simulink model "CONTROLADORES"  (R2018b)
settings: Solver=VariableStepAuto  StartTime=0.0  StopTime=8  RelTol=1e-3
undefined symbols (not defined in the file or in its folder): DiscIntNeverNeededParam, Gp, Gp_ps, M1p, magnitude, PID_Z, PIDM1z, Ts
libraries: simulink x3
settings Model: Creator=Vflrz17  LastModifiedBy=Atomauro
settings SFSimCC: SimUseLocalCustomCode=off
settings RTWCC: RTWUseLocalCustomCode=off

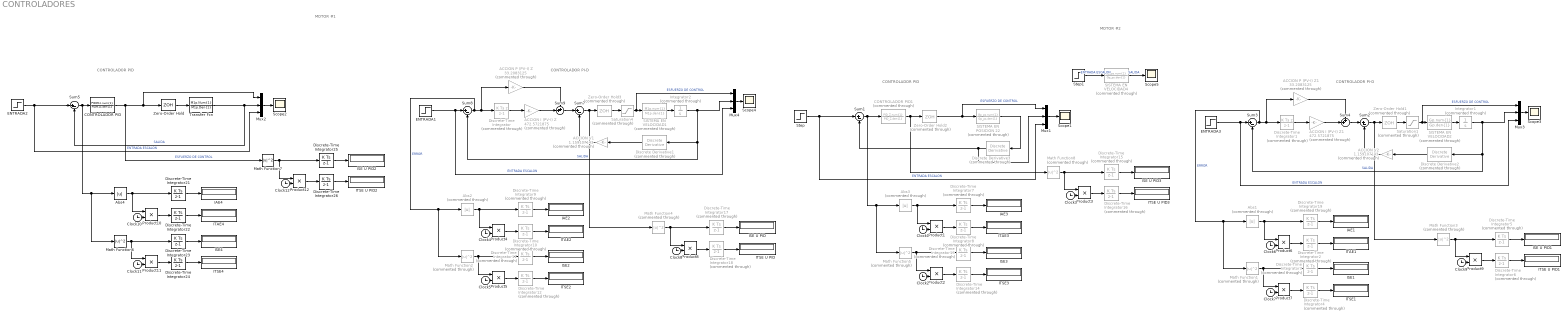
== system CONTROLADORES ==
  note: MOTOR #1
  note: CONTROLADOR PID
  note: CONTROLADOR PI-D
  note: MOTOR #2
  note: CONTROLADOR PID
  note: CONTROLADOR PI-D
  ACCION I (PV-I) Z : Gain  Commented=through  Gain=472.5721875
  ACCION I (PV-I) Z1 : Gain  Commented=through  Gain=472.5721875
  ACCION P (PV-I) Z : Gain  Commented=through  Gain=33.2083125
  ACCION P (PV-I) Z1 : Gain  Commented=through  Gain=33.2083125
  ACCION V1 : Gain  Commented=through  Gain=1.159107143
  ACCION V2 : Gain  Commented=through  Gain=1.159107143
  Abs1 : Abs  Commented=through
  Abs2 : Abs  Commented=through
  Abs3 : Abs  Commented=through
  Abs4 : Abs
  CONTROLADOR PID : DiscreteTransferFcn  Numerator=PIDM1z.num{1}  Denominator=PIDM1z.den{1}  SampleTime=Ts
  CONTROLADOR PID1 : DiscreteTransferFcn  Commented=through  Numerator=PID_Z.num{1}  Denominator=PID_Z.den{1}  SampleTime=Ts
  Clock{1..12} (12 alike) : Clock
  Discrete Derivative1 : simulink/Discrete/Discrete Derivative  Commented=through  gainval=1.0  ICPrevScaledInput=0.0  OutMin=[]  OutMax=[]  OutDataType=fixdt(1, 16)  OutScaling=2^-10  DoSatur=off
  Discrete Derivative2 : simulink/Discrete/Discrete Derivative  Commented=through  gainval=1.0  ICPrevScaledInput=0.0  OutMin=[]  OutMax=[]  OutDataType=fixdt(1, 16)  OutScaling=2^-10  DoSatur=off
  Discrete Derivative3 : simulink/Discrete/Discrete Derivative  Commented=through  gainval=1.0  ICPrevScaledInput=0.0  OutMin=[]  OutMax=[]  OutDataType=fixdt(1, 16)  OutScaling=2^-10  DoSatur=off
  Discrete-Time Integrator : DiscreteIntegrator  Commented=through  IntegratorMethod=Integration: Backward Euler  gainval=1  SampleTime=0.1  ICPrevOutput=DiscIntNeverNeededParam  ICPrevScaledInput=DiscIntNeverNeededParam
  Discrete-Time Integrator1 : DiscreteIntegrator  Commented=through  IntegratorMethod=Integration: Backward Euler  gainval=1  SampleTime=0.1  ICPrevOutput=DiscIntNeverNeededParam  ICPrevScaledInput=DiscIntNeverNeededParam
  Discrete-Time Integrator{2..19} (18 alike) : DiscreteIntegrator  Commented=through  gainval=1  SampleTime=Ts  ICPrevOutput=DiscIntNeverNeededParam  ICPrevScaledInput=DiscIntNeverNeededParam
  Discrete-Time Integrator{21..26} (6 alike) : DiscreteIntegrator  gainval=1  SampleTime=Ts  ICPrevOutput=DiscIntNeverNeededParam  ICPrevScaledInput=DiscIntNeverNeededParam
  ENTRADA1 : Step  SampleTime=0
  ENTRADA2 : Step  SampleTime=0
  ENTRADA3 : Step  SampleTime=Ts
  IAE{1..4} (4 alike) : Display
  ISE U PID{,1..3} (4 alike) : Display
  ISE{1..4} (4 alike) : Display
  ITAE{1..4} (4 alike) : Display
  ITSE U PID{,1..3} (4 alike) : Display
  ITSE{1..4} (4 alike) : Display
  Integrator1 : Integrator  Commented=through
  Integrator2 : Integrator  Commented=through
  Math Function{1..5,8} (6 alike) : Math  Commented=through  Operator=magnitude^2  SaturateOnIntegerOverflow=on
  Math Function6 : Math  Operator=magnitude^2  SaturateOnIntegerOverflow=on
  Math Function7 : Math  Operator=magnitude^2  SaturateOnIntegerOverflow=on
  Mux{1..4} (4 alike) : Mux  Inputs=3
  Product{1..12} (12 alike) : Product
  SISTEMA EN POSICION 22 : TransferFcn  Commented=through  Numerator=Gp_ps.num{1}  Denominator=Gp_ps.den{1}
  SISTEMA EN VELOCIDAD1 : TransferFcn  Commented=through  Numerator=M1p.num{1}  Denominator=M1p.den{1}
  SISTEMA EN VELOCIDAD2 : TransferFcn  Commented=through  Numerator=Gp.num{1}  Denominator=Gp.den{1}
  SISTEMA EN VELOCIDAD4 : TransferFcn  Commented=through  Numerator=Gp_ps.num{1}  Denominator=Gp_ps.den{1}
  Saturation1 : Saturate  Commented=through  UpperLimit=10  LowerLimit=-10
  Saturation4 : Saturate  Commented=through  UpperLimit=10  LowerLimit=-10
  Scope{1..5} (5 alike) : Scope
  Step : Step  SampleTime=0
  Step1 : Step  SampleTime=0
  Sum{1..3,5,7..8} (6 alike) : Sum  Inputs=|+-
  Sum4 : Sum  Inputs=++|
  Sum9 : Sum  Inputs=++|
  Transfer Fcn : TransferFcn  Numerator=M1p.Num{1}  Denominator=M1p.Den{1}
  Zero-Order Hold : ZeroOrderHold  SampleTime=-1
  Zero-Order Hold1 : ZeroOrderHold  Commented=through  SampleTime=Ts
  Zero-Order Hold2 : ZeroOrderHold  Commented=through  SampleTime=Ts
  Zero-Order Hold3 : ZeroOrderHold  Commented=through  SampleTime=-1
  wires:
  Mux2/1 -> Scope2/1
  ENTRADA2/1 -> Sum5/1, Mux2/3  "ENTRADA ESCALON"
  Transfer Fcn/1 -> Sum5/2, Mux2/2  "SALIDA"
  CONTROLADOR PID/1 -> Zero-Order Hold/1, Mux2/1, Math Function7/1  "ESFUERZO DE CONTROL"
  Clock12/1 -> Product12/2
  Product12/1 -> Discrete-Time Integrator26/1
  Discrete-Time Integrator24/1 -> ITSE4/1
  Discrete-Time Integrator26/1 -> ITSE U PID2/1
  Math Function7/1 -> Discrete-Time Integrator25/1, Product12/1
  Discrete-Time Integrator25/1 -> ISE U PID2/1
  Abs4/1 -> Product10/1, Discrete-Time Integrator21/1
  Discrete-Time Integrator21/1 -> IAE4/1
  Product11/1 -> Discrete-Time Integrator24/1
  Clock10/1 -> Product10/2
  Sum5/1 -> Abs4/1, Math Function6/1, CONTROLADOR PID/1
  Discrete-Time Integrator22/1 -> ITAE4/1
  Product10/1 -> Discrete-Time Integrator22/1
  Math Function6/1 -> Discrete-Time Integrator23/1, Product11/1
  Clock11/1 -> Product11/2
  Discrete-Time Integrator23/1 -> ISE4/1
  Discrete-Time Integrator12/1 -> ITSE2/1
  Clock5/1 -> Product5/2
  Sum8/1 -> Abs2/1, Math Function2/1, Discrete-Time Integrator/1, ACCION P (PV-I) Z/1  "ERROR"
  Product8/1 -> Discrete-Time Integrator18/1
  Saturation4/1 -> Mux4/1, SISTEMA EN VELOCIDAD1/1  "ESFUERZO DE CONTROL"
  Abs2/1 -> Product4/1, Discrete-Time Integrator9/1
  Mux4/1 -> Scope4/1
  Sum7/1 -> Math Function4/1, Zero-Order Hold3/1
  ACCION P (PV-I) Z/1 -> Sum9/1
  ENTRADA1/1 -> Mux4/3, Sum8/1  "ENTRADA ESCALON"
  Discrete Derivative1/1 -> ACCION V1/1
  Sum9/1 -> Sum7/1
  Product4/1 -> Discrete-Time Integrator10/1
  SISTEMA EN VELOCIDAD1/1 -> Integrator2/1
  Discrete-Time Integrator18/1 -> ITSE U PID/1
  Integrator2/1 -> Mux4/2, Discrete Derivative1/1, Sum8/2  "SALIDA"
  Discrete-Time Integrator9/1 -> IAE2/1
  ACCION I (PV-I) Z/1 -> Sum9/2
  Math Function2/1 -> Discrete-Time Integrator11/1, Product5/1
  ACCION V1/1 -> Sum7/2
  Discrete-Time Integrator10/1 -> ITAE2/1
  Discrete-Time Integrator17/1 -> ISE U PID/1
  Clock8/1 -> Product8/2
  Product5/1 -> Discrete-Time Integrator12/1
  Clock4/1 -> Product4/2
  Discrete-Time Integrator11/1 -> ISE2/1
  Zero-Order Hold3/1 -> Saturation4/1
  Math Function4/1 -> Discrete-Time Integrator17/1, Product8/1
  Discrete-Time Integrator/1 -> ACCION I (PV-I) Z/1
  Discrete-Time Integrator1/1 -> ACCION I (PV-I) Z1/1
  Math Function3/1 -> Product9/1, Discrete-Time Integrator5/1
  Zero-Order Hold1/1 -> Saturation1/1
  Discrete-Time Integrator3/1 -> ISE1/1
  Clock6/1 -> Product6/2
  Product7/1 -> Discrete-Time Integrator4/1
  Clock9/1 -> Product9/2
  Discrete-Time Integrator5/1 -> ISE U PID1/1
  Discrete-Time Integrator2/1 -> ITAE1/1
  ACCION V2/1 -> Sum2/2
  Math Function1/1 -> Product7/1, Discrete-Time Integrator3/1
  ACCION I (PV-I) Z1/1 -> Sum4/2
  Discrete-Time Integrator19/1 -> IAE1/1
  Integrator1/1 -> Sum3/2, Discrete Derivative2/1, Mux3/2  "SALIDA"
  Discrete-Time Integrator6/1 -> ITSE U PID1/1
  SISTEMA EN VELOCIDAD2/1 -> Integrator1/1
  Product6/1 -> Discrete-Time Integrator2/1
  Sum4/1 -> Sum2/1
  Discrete Derivative2/1 -> ACCION V2/1
  ENTRADA3/1 -> Sum3/1, Mux3/3  "ENTRADA ESCALON"
  ACCION P (PV-I) Z1/1 -> Sum4/1
  Sum2/1 -> Zero-Order Hold1/1, Math Function3/1
  Mux3/1 -> Scope3/1
  Abs1/1 -> Discrete-Time Integrator19/1, Product6/1
  Saturation1/1 -> SISTEMA EN VELOCIDAD2/1, Mux3/1  "ESFUERZO DE CONTROL"
  Product9/1 -> Discrete-Time Integrator6/1
  Sum3/1 -> ACCION P (PV-I) Z1/1, Discrete-Time Integrator1/1, Math Function1/1, Abs1/1  "ERROR"
  Clock7/1 -> Product7/2
  Discrete-Time Integrator4/1 -> ITSE1/1
  Discrete-Time Integrator13/1 -> ISE3/1
  Clock2/1 -> Product2/2
  Math Function5/1 -> Product2/1, Discrete-Time Integrator13/1
  Product1/1 -> Discrete-Time Integrator8/1
  Discrete-Time Integrator8/1 -> ITAE3/1
  Sum1/1 -> CONTROLADOR PID1/1, Math Function5/1, Abs3/1
  Clock1/1 -> Product1/2
  Product2/1 -> Discrete-Time Integrator14/1
  Discrete-Time Integrator7/1 -> IAE3/1
  Abs3/1 -> Discrete-Time Integrator7/1, Product1/1
  Discrete-Time Integrator15/1 -> ISE U PID3/1
  Math Function8/1 -> Product3/1, Discrete-Time Integrator15/1
  Discrete-Time Integrator16/1 -> ITSE U PID3/1
  Discrete-Time Integrator14/1 -> ITSE3/1
  Product3/1 -> Discrete-Time Integrator16/1
  Clock3/1 -> Product3/2
  CONTROLADOR PID1/1 -> Math Function8/1, Zero-Order Hold2/1
  Step/1 -> Mux1/3, Sum1/1  "ENTRADA ESCALON"
  Mux1/1 -> Scope1/1
  Zero-Order Hold2/1 -> SISTEMA EN POSICION 22/1, Mux1/1  "ESFUERZO DE CONTROL"
  SISTEMA EN POSICION 22/1 -> Discrete Derivative3/1
  Step1/1 -> SISTEMA EN VELOCIDAD4/1  "ENTRADA ESCALON"
  SISTEMA EN VELOCIDAD4/1 -> Scope5/1  "SALIDA"
  Discrete Derivative3/1 -> Mux1/2, Sum1/2
  Zero-Order Hold/1 -> Transfer Fcn/1
